simulink model "main"  (R2024a)
settings: Solver=FixedStepAuto  StartTime=0.0  StopTime=10  FixedStep=0.01  RelTol=1e-3
values from neighbouring files (symbols this model uses):
  denom_tf = (conv(mech,elec)+Kt*Kb)    [transfer_fn.m]
  kd = 10    [transfer_fn.m]
  ki = 100    [transfer_fn.m]
  kp = 150    [transfer_fn.m]
  num_tf = Kt    (= 0.01)    [transfer_fn.m]
libraries: spspowerguiLib x1
settings Model: Creator=farza  LastModifiedBy=farza

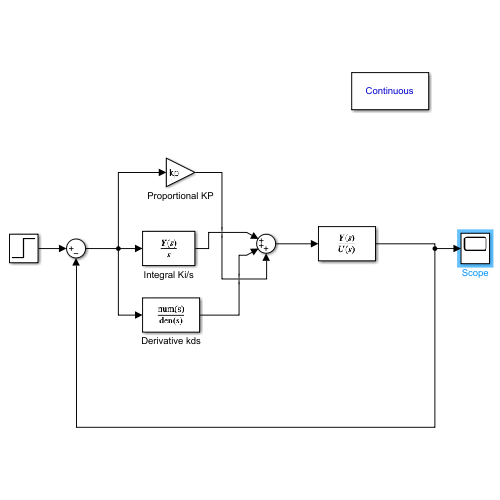
[thumbnail: Simulink's stored preview of the top-level diagram]
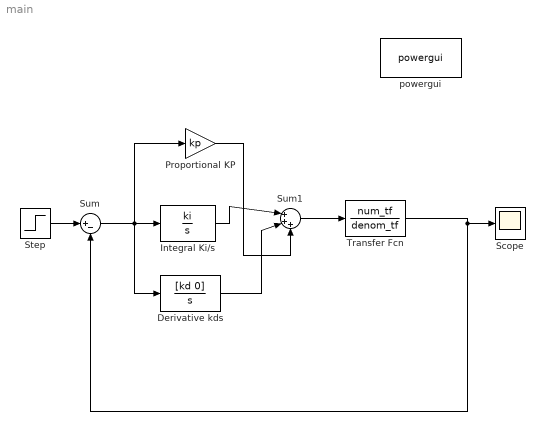
== system main ==
  Derivative kds : TransferFcn  Numerator=[kd 0]  Denominator=[1 0]
  Integral Ki/s : TransferFcn  Numerator=ki  Denominator=[1 0]
  Proportional KP : Gain  Gain=kp
  Scope : Scope
  Step : Step  After=100  SampleTime=0
  Sum : Sum  Inputs=|+-
  Sum1 : Sum  Inputs=|+++
  Transfer Fcn : TransferFcn  Numerator=num_tf  Denominator=denom_tf
  powergui : spspowerguiLib/powergui  Priority=1  SimulationMode=Continuous  SampleTime=50e-6  frequency=60  Iterations=50  frequencyindice=60  Pbase=100e6  ErrMax=1e-4  UnitsV=kV  UnitsW=MW  buscounter=0  FunctionMessages=off  echomessages=off  EnableUseOfTLC=off  CurrentSourceSwitches=off  DisableSnubberDevices=off  DisableRonSwitches=off  DisableVfSwitches=off  DisplayEquations=off  AutomaticDiscreteSolvers=off  SolverType=Tustin/Backward Euler (TBE)  Interpol=off  ExternalGateDelay=off  methode=off  Ts=100  x0status=blocks  SPID=on  SwTol=0  HookPort=off  NonlinearTolerance=1e-4  nMaxIteration=100  ContinueOnMaxIteration=off  RestoreLinks=warning  ResistiveCurrentMeasurement=off  Frange=[0:2:500]  Ylog=off  Xlog=on  ShowGrid=off  save=off  variable=ZData  structure=0  ZoomFFT=off  StartTime=0.0  cycles=1  DisplayStyle=1  fundamental=60  FreqAxis=off  MaxFrequency=1000  frequencyindicesteady=1  RmsSteady=1  display=off
  wires:
  Step/1 -> Sum/1
  Sum/1 -> Derivative kds/1, Integral Ki/s/1, Proportional KP/1
  Transfer Fcn/1 -> Sum/2, Scope/1
  Integral Ki/s/1 -> Sum1/1
  Derivative kds/1 -> Sum1/2
  Proportional KP/1 -> Sum1/3
  Sum1/1 -> Transfer Fcn/1
